simulink model "F2sidecarv4"  (R2018b)
settings: Solver=ode45  StartTime=0.0  StopTime=20  MaxStep=1e-3  RelTol=1e-5
values from neighbouring files (symbols this model uses):
  g = 9.8    [GG.m]    (also in main.m)
  HGC = 0.165    [main.m]
  Iz = 80    [main.m]
  lf = 0.7    [main.m]
  lr = WB-lf    (= 0.6)    [main.m]
  ls = lr-lshift    (= 0.6)    [main.m]
  lshift = 0.2    [main.m]
  m = 180    [main.m]
  TrackL = 0.7*Track    (= 0.7735)    [main.m]
  TrackRf = TrackRr-frontwheel_shift    (= 0.3315)    [main.m]
  TrackRr = Track-TrackL    (= 0.3315)    [main.m]
  v0 = 20    [main.m]
  WB = 1.2    [main.m]
libraries: simulink x5
settings Model: Creator=PHADM  LastModifiedBy=PHADM
settings SolverCC: AlgebraicLoopSolver=LineSearch

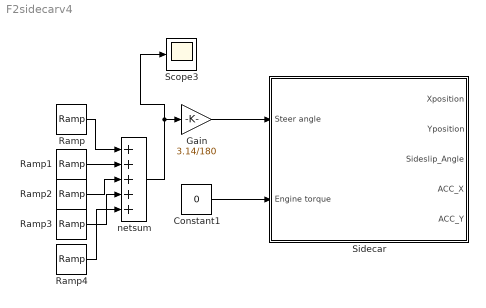
== system F2sidecarv4 ==
  Constant1 : Constant  Value=0
  Gain : Gain  Gain=3.14/180
  Ramp : simulink/Sources/Ramp  slope=-10  start=0  InitialOutput=0
  Ramp1 : simulink/Sources/Ramp  slope=10  start=2  InitialOutput=0
  Ramp2 : simulink/Sources/Ramp  slope=0  start=3  InitialOutput=0
  Ramp3 : simulink/Sources/Ramp  slope=0  start=8  InitialOutput=0
  Ramp4 : simulink/Sources/Ramp  slope=0  start=10  InitialOutput=0
  Scope3 : Scope
  "Sidecar " : Subsystem
  netsum : Sum  Inputs=5  SaturateOnIntegerOverflow=on  InputSameDT=on  OutDataTypeStr=Inherit: Same as first input
  wires:
  Constant1/1 -> "Sidecar "/2(Engine torque)
  Gain/1 -> "Sidecar "/1("Steer angle ")
  Ramp/1 -> netsum/1
  netsum/1 -> Scope3/1, Gain/1
  Ramp1/1 -> netsum/2
  Ramp2/1 -> netsum/3
  Ramp3/1 -> netsum/4
  Ramp4/1 -> netsum/5

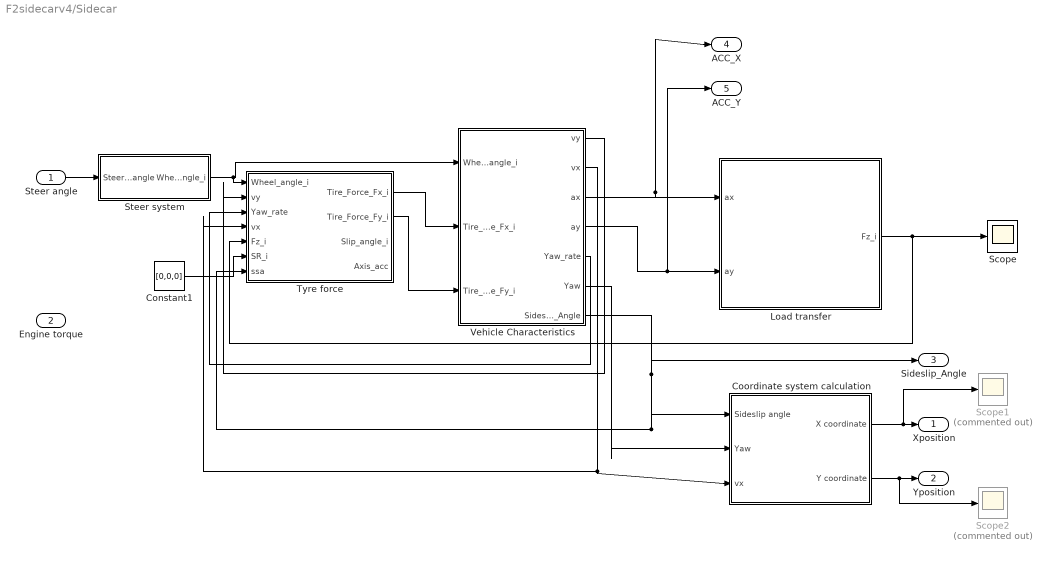
== system F2sidecarv4/Sidecar  ==
  "Steer angle " : Inport
  Engine torque : Inport  Port=2
  Constant1 : Constant  Value=[0,0,0]
  Coordinate system calculation : Subsystem
  Load transfer : Subsystem
  Scope : Scope
  Scope1 : Scope  Commented=on
  Scope2 : Scope  Commented=on
  Steer system : Subsystem
  Tyre force : Subsystem
  Vehicle Characteristics : Subsystem
  Xposition : Outport
  Yposition : Outport  Port=2
  Sideslip_Angle : Outport  Port=3
  ACC_X : Outport  Port=4
  ACC_Y : Outport  Port=5
  wires:
  Steer system/1(Wheel_angle_i) -> Vehicle Characteristics/1(Wheel_angle_i), Tyre force/1(Wheel_angle_i)
  Vehicle Characteristics/3(ax) -> ACC_X/1, Load transfer/1(ax)
  Vehicle Characteristics/4(ay) -> ACC_Y/1, Load transfer/2(ay)
  Vehicle Characteristics/6(Yaw) -> Coordinate system calculation/2(Yaw)
  Vehicle Characteristics/2(vx) -> Tyre force/4(vx), Coordinate system calculation/3(vx)
  Coordinate system calculation/1(X coordinate) -> Scope1/1, Xposition/1
  Coordinate system calculation/2(Y coordinate) -> Scope2/1, Yposition/1
  Tyre force/1(Tire_Force_Fx_i) -> Vehicle Characteristics/2("Tire_Force_Fx_i ")
  Tyre force/2(Tire_Force_Fy_i) -> Vehicle Characteristics/3(Tire_Force_Fy_i)
  Constant1/1 -> Tyre force/6(SR_i)
  Vehicle Characteristics/5(Yaw_rate) -> Tyre force/3(Yaw_rate)
  Vehicle Characteristics/7(Sideslip_Angle) -> Coordinate system calculation/1(Sideslip angle), Tyre force/7(ssa), Sideslip_Angle/1
  Load transfer/1(Fz_i) -> Tyre force/5(Fz_i), Scope/1
  Vehicle Characteristics/1(vy) -> Tyre force/2(vy)
  "Steer angle "/1 -> Steer system/1(Steer_angle)

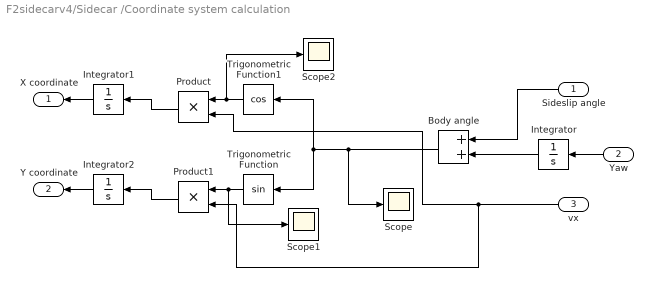
== system F2sidecarv4/Sidecar /Coordinate system calculation ==
  Sideslip angle : Inport
  Yaw : Inport  Port=2
  vx : Inport  Port=3
  Body angle : Sum
  Integrator : Integrator
  Integrator1 : Integrator
  Integrator2 : Integrator
  Product : Product
  Product1 : Product
  Scope : Scope
  Scope1 : Scope
  Scope2 : Scope
  Trigonometric Function : Trigonometry
  Trigonometric Function1 : Trigonometry  Operator=cos
  X coordinate : Outport
  Y coordinate : Outport  Port=2
  wires:
  vx/1 -> Product/2, Product1/2
  Yaw/1 -> Integrator/1
  Sideslip angle/1 -> Body angle/1
  Integrator2/1 -> Y coordinate/1
  Integrator1/1 -> X coordinate/1
  Product1/1 -> Integrator2/1
  Product/1 -> Integrator1/1
  Trigonometric Function/1 -> Scope1/1, Product1/1
  Trigonometric Function1/1 -> Product/1, Scope2/1
  Body angle/1 -> Scope/1, Trigonometric Function1/1, Trigonometric Function/1
  Integrator/1 -> Body angle/2

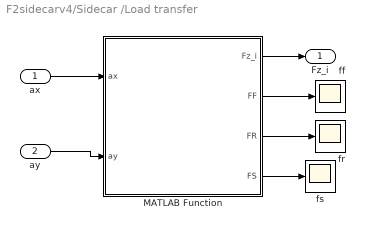
== system F2sidecarv4/Sidecar /Load transfer ==
  ax : Inport
  ay : Inport  Port=2
  MATLAB Function : MATLAB Function  TreatAsAtomicUnit=on
  ff : Scope
  fr : Scope
  fs : Scope
  Fz_i : Outport
  wires:
  MATLAB Function/1(Fz_i) -> Fz_i/1
  ax/1 -> MATLAB Function/1(ax)
  ay/1 -> MATLAB Function/2(ay)
  MATLAB Function/4(FS) -> fs/1
  MATLAB Function/3(FR) -> fr/1
  MATLAB Function/2(FF) -> ff/1

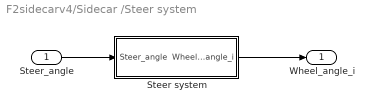
== system F2sidecarv4/Sidecar /Steer system ==
  Steer_angle : Inport
  Steer system : MATLAB Function  TreatAsAtomicUnit=on
  Wheel_angle_i : Outport
  wires:
  Steer_angle/1 -> Steer system/1(Steer_angle)
  Steer system/1(Wheel_angle_i) -> Wheel_angle_i/1

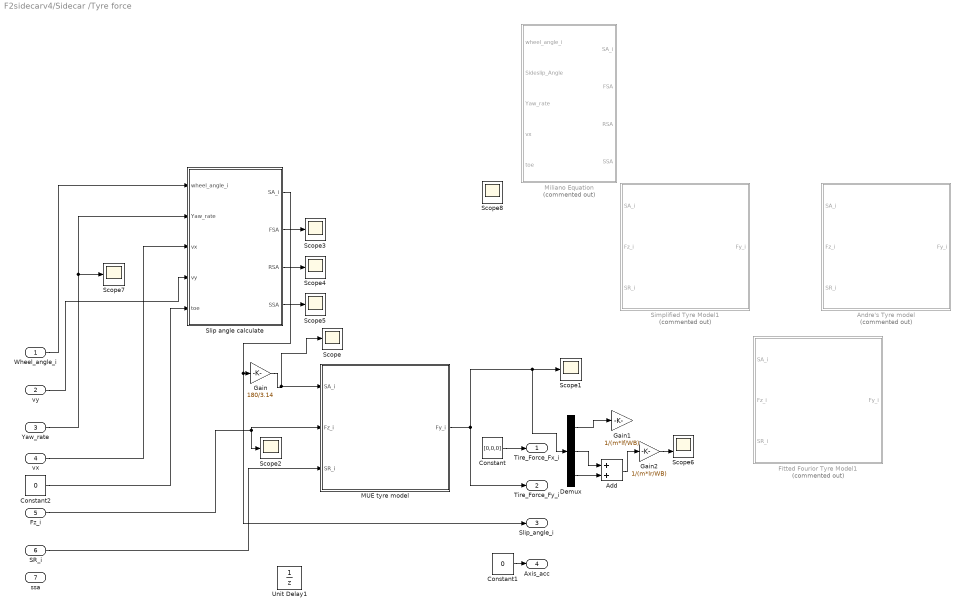
== system F2sidecarv4/Sidecar /Tyre force ==
  Wheel_angle_i : Inport
  vy : Inport  Port=2
  Yaw_rate : Inport  Port=3
  vx : Inport  Port=4
  Fz_i : Inport  Port=5
  SR_i : Inport  Port=6
  ssa : Inport  Port=7
  Add : Sum
  Andre's Tyre model : MATLAB Function  Commented=on  TreatAsAtomicUnit=on
  Constant : Constant  Value=[0,0,0]
  Constant1 : Constant  Value=0
  Constant2 : Constant  Value=0
  Demux : Demux  Outputs=3
  Fitted Fourior Tyre Model1 : MATLAB Function  Commented=on  TreatAsAtomicUnit=on
  Gain : Gain  Gain=180/3.14
  Gain1 : Gain  Gain=1/(m*lf/WB)
  Gain2 : Gain  Gain=1/(m*lr/WB)
  MUE tyre model : MATLAB Function  TreatAsAtomicUnit=on
  Miliano Equation : MATLAB Function  Commented=on  TreatAsAtomicUnit=on
  Scope{,1..5,7..8} (8 alike) : Scope
  Scope6 : Scope  NumInputPorts=2
  Simplified Tyre Model1 : MATLAB Function  Commented=on  TreatAsAtomicUnit=on
  Slip angle calculate : MATLAB Function  TreatAsAtomicUnit=on
  Unit Delay1 : UnitDelay  SampleTime=-1
  Tire_Force_Fx_i : Outport
  Tire_Force_Fy_i : Outport  Port=2
  Slip_angle_i : Outport  Port=3
  Axis_acc : Outport  Port=4
  wires:
  Wheel_angle_i/1 -> Slip angle calculate/1(wheel_angle_i)
  vy/1 -> Slip angle calculate/4(vy)
  Yaw_rate/1 -> Slip angle calculate/2(Yaw_rate), Scope7/1
  vx/1 -> Slip angle calculate/3(vx)
  Constant/1 -> Tire_Force_Fx_i/1
  Constant1/1 -> Axis_acc/1
  SR_i/1 -> MUE tyre model/3(SR_i)
  MUE tyre model/1(Fy_i) -> Demux/1, Scope1/1, Tire_Force_Fy_i/1
  Constant2/1 -> Slip angle calculate/5(toe)
  Slip angle calculate/2(FSA) -> Scope3/1
  Slip angle calculate/3(RSA) -> Scope4/1
  Slip angle calculate/4(SSA) -> Scope5/1
  Fz_i/1 -> MUE tyre model/2(Fz_i), Scope2/1
  Gain/1 -> MUE tyre model/1(SA_i), Scope/1
  Demux/1 -> Gain1/1
  Demux/2 -> Add/1
  Gain2/1 -> Scope6/2
  Demux/3 -> Add/2
  Add/1 -> Gain2/1
  Slip angle calculate/1(SA_i) -> Slip_angle_i/1, Gain/1

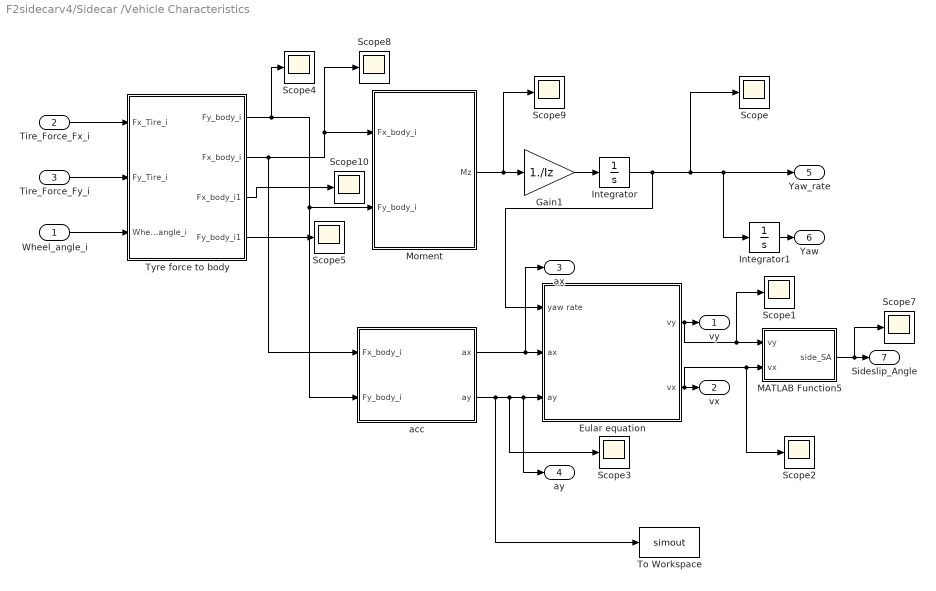
== system F2sidecarv4/Sidecar /Vehicle Characteristics ==
  Wheel_angle_i : Inport
  "Tire_Force_Fx_i " : Inport  Port=2
  Tire_Force_Fy_i : Inport  Port=3
  Eular equation : Subsystem
  Gain1 : Gain  Gain=1./Iz
  Integrator : Integrator
  Integrator1 : Integrator
  MATLAB Function5 : MATLAB Function  TreatAsAtomicUnit=on
  Moment : MATLAB Function  TreatAsAtomicUnit=on
  Scope{,1..5,7..10} (10 alike) : Scope
  To Workspace : ToWorkspace  VariableName=simout  SaveFormat=Timeseries  SampleTime=-1
  Tyre force to body : Subsystem
  acc : MATLAB Function  TreatAsAtomicUnit=on
  vy : Outport
  vx : Outport  Port=2
  ax : Outport  Port=3
  ay : Outport  Port=4
  Yaw_rate : Outport  Port=5
  Yaw : Outport  Port=6
  Sideslip_Angle : Outport  Port=7
  wires:
  Wheel_angle_i/1 -> Tyre force to body/3(Wheel_angle_i)
  Tire_Force_Fy_i/1 -> Tyre force to body/2(Fy_Tire_i)
  "Tire_Force_Fx_i "/1 -> Tyre force to body/1(Fx_Tire_i)
  Moment/1(Mz) -> Scope9/1, Gain1/1
  Gain1/1 -> Integrator/1
  Integrator/1 -> Eular equation/1(yaw rate), Integrator1/1, Yaw_rate/1, Scope/1
  Integrator1/1 -> Yaw/1
  acc/1(ax) -> ax/1, Eular equation/2(ax)
  acc/2(ay) -> To Workspace/1, Scope3/1, ay/1, Eular equation/3(ay)
  Eular equation/1(vy) -> Scope1/1, MATLAB Function5/1(vy), vy/1
  Eular equation/2(vx) -> Scope2/1, MATLAB Function5/2(vx), vx/1
  MATLAB Function5/1(side_SA) -> Scope7/1, Sideslip_Angle/1
  Tyre force to body/1(Fy_body_i) -> Scope4/1, acc/2(Fy_body_i), Moment/2(Fy_body_i)
  Tyre force to body/4(Fy_body_i1) -> Scope5/1
  Tyre force to body/2(Fx_body_i) -> acc/1(Fx_body_i), Moment/1(Fx_body_i), Scope8/1
  Tyre force to body/3(Fx_body_i1) -> Scope10/1

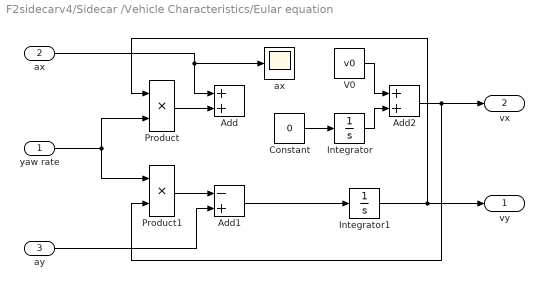
== system F2sidecarv4/Sidecar /Vehicle Characteristics/Eular equation ==
  yaw rate : Inport
  ax : Inport  Port=2
  ay : Inport  Port=3
  Add : Sum
  Add1 : Sum  Inputs=-+
  Add2 : Sum
  Constant : Constant  Value=0
  Integrator : Integrator  LimitOutput=on  LowerSaturationLimit=0  IgnoreLimit=on
  Integrator1 : Integrator  LowerSaturationLimit=0  IgnoreLimit=on
  Product : Product
  Product1 : Product
  V0 : Constant  Value=v0
  "ax " : Scope
  vy : Outport
  vx : Outport  Port=2
  wires:
  yaw rate/1 -> Product/2, Product1/1
  ax/1 -> "ax "/1, Add/1
  Add1/1 -> Integrator1/1
  Integrator/1 -> Add2/2
  Product1/1 -> Add1/1
  ay/1 -> Add1/2
  Constant/1 -> Integrator/1
  V0/1 -> Add2/1
  Integrator1/1 -> vy/1, Product/1
  Product/1 -> Add/2
  Add2/1 -> Product1/2, vx/1

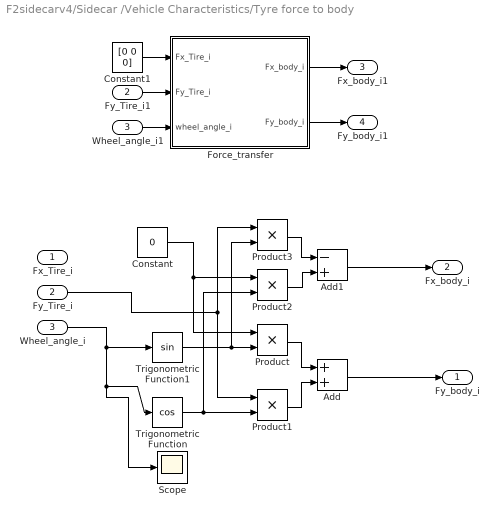
== system F2sidecarv4/Sidecar /Vehicle Characteristics/Tyre force to body ==
  Fx_Tire_i : Inport
  Fy_Tire_i : Inport  Port=2
  Wheel_angle_i : Inport  Port=3
  Add : Sum
  Add1 : Sum  Inputs=-+
  Constant : Constant  Value=0
  Constant1 : Constant  Value=[0 0 0]
  Force_transfer : MATLAB Function  TreatAsAtomicUnit=on
  Fy_Tire_i1 : InportShadow  Port=2
  Product{,1..3} (4 alike) : Product
  Scope : Scope
  Trigonometric Function : Trigonometry  Operator=cos  ApproximationMethod=CORDIC
  Trigonometric Function1 : Trigonometry  ApproximationMethod=CORDIC
  Wheel_angle_i1 : InportShadow  Port=3
  Fy_body_i : Outport
  Fx_body_i : Outport  Port=2
  Fx_body_i1 : Outport  Port=3
  Fy_body_i1 : Outport  Port=4
  wires:
  Constant/1 -> Product/1, Product2/1
  Product2/1 -> Add1/2
  Product3/1 -> Add1/1
  Product1/1 -> Add/2
  Product/1 -> Add/1
  Fy_Tire_i/1 -> Product1/1, Product3/1
  Trigonometric Function/1 -> Product1/2, Product2/2
  Trigonometric Function1/1 -> Product/2, Product3/2
  Wheel_angle_i/1 -> Scope/1, Trigonometric Function/1, Trigonometric Function1/1
  Add1/1 -> Fx_body_i/1
  Add/1 -> Fy_body_i/1
  Force_transfer/2(Fy_body_i) -> Fy_body_i1/1
  Force_transfer/1(Fx_body_i) -> Fx_body_i1/1
  Fy_Tire_i1/1 -> Force_transfer/2(Fy_Tire_i)
  Constant1/1 -> Force_transfer/1(Fx_Tire_i)
  Wheel_angle_i1/1 -> Force_transfer/3(wheel_angle_i)

== matlab function F2sidecarv4/Sidecar /Tyre force/Fitted Fourior Tyre Model1 ==
  data: SA_i input size=3; Fy_i output size=3; Fz_i input size=3; SR_i input size=3
function Fy_i = fcn(SA_i,Fz_i,SR_i)
SR_i=[0,0,0];
Fy_i=zeros(3,1);
Fy_i0=zeros(3,1);


i=1;
while i<4
    if SA_i(i)>10
    SA_i(i)=10;
else if SA_i(i)<-10
        SA_i(i)=-10;
    end
end
Fy_i0(i)=  -85.64 + 115*cos(SA_i(i)*0.3621) + 1640*sin(SA_i(i)*0.3621) + (-117.5)*cos(2*SA_i(i)*0.3621) + (-158.2)*sin(2*SA_i(i)*0.3621) + 70.39*cos(3*SA_i(i)*0.3621) + 221.5*sin(3*SA_i(i)*0.3621) +(-50.6)*cos(4*SA_i(i)*0.3621) + (-14.42)*sin(4*SA_i(i)*0.3621) + 19.82*cos(5*SA_i(i)*0.3621) + 20.98*sin(5*SA_i(i)*0.3621) + (-8.731)*cos(6*SA_i(i)*0.3621) + 9.067*sin(6*SA_i(i)*0.3621);
Fy_i(i)=0.65*Fy_i0(i);
i=i+1;
end
end

== matlab function F2sidecarv4/Sidecar /Tyre force/Miliano Equation ==
  data: wheel_angle_i input; SA_i output; Sideslip_Angle input; Yaw_rate input; vx input; FSA output; RSA output; SSA output; lf parameter; lr parameter; lshift parameter; TrackL parameter; TrackRf parameter; toe input; TrackRr parameter
%%TrackL+TrackR=Track
%%lr+lf=Wheel base
%%ls-distance gravity centre to sidewheel
function [SA_i,FSA,RSA,SSA] = fcn(wheel_angle_i,Sideslip_Angle,Yaw_rate,vx,lf, lr, lshift, TrackL, TrackRf,toe, TrackRr)
SA_i=zeros(3,1);

SA_i(1)=atan(((vx*tan(Sideslip_Angle)+Yaw_rate*lf)*cos(wheel_angle_i(1))-((vx-Yaw_rate*TrackRf)*cos(wheel_angle_i(1))))/((vx-Yaw_rate*TrackRf)*cos(wheel_angle_i(1))+(vx*tan(Sideslip_Angle)+Yaw_rate*lf)*sin(wheel_angle_i(1)))); %%front wheel(right)
SA_i(2)=atan((vx*tan(Sideslip_Angle)-Yaw_rate*lr)/(vx+Yaw_rate*TrackRr));%%rear wheel(right)
SA_i(3)=atan(((vx*tan(Sideslip_Angle)-Yaw_rate*(lshift))*cos(toe)-(vx-Yaw_rate*(TrackL))*sin(toe))/(vx-Yaw_rate*(TrackL)*cos(toe)+(vx*tan(Sideslip_Angle)+Yaw_rate*(lshift)))); %%side wheel(left)

FSA=SA_i(1);
RSA=SA_i(2);
SSA=SA_i(3);
end

== matlab function F2sidecarv4/Sidecar /Steer system/Steer system ==
  data: Steer_angle input; Wheel_angle_i output
function Wheel_angle_i  = fcn(Steer_angle)
Wheel_angle_i=zeros(3,1);
Wheel_angle_i(1) = Steer_angle;
Wheel_angle_i(2)=0;
Wheel_angle_i(3)=0;
end

== matlab function F2sidecarv4/Sidecar /Vehicle Characteristics/Moment ==
  data: Fx_body_i input size=3; Mz output; Fy_body_i input size=3; lf parameter; lr parameter; ls parameter; TrackL parameter; TrackRf parameter; TrackRr parameter
function Mz = fcn(Fx_body_i,Fy_body_i,lf, lr, ls, TrackL, TrackRf,TrackRr)
Mz=zeros(1,1);
Mz=Fy_body_i(1).*lf-Fy_body_i(2).*lr-Fy_body_i(3).*ls+TrackRf*(-(Fx_body_i(1)))+TrackRr*(-(Fx_body_i(2))+TrackL*(Fx_body_i(3)));
end

== matlab function F2sidecarv4/Sidecar /Vehicle Characteristics/acc ==
  data: Fx_body_i input size=3; ax output; Fy_body_i input size=3; ay output; m parameter
function [ax,ay] = fcn(Fx_body_i,Fy_body_i,m)

ax=(Fx_body_i(1)+Fx_body_i(2)+Fx_body_i(3))/m;
ay=(Fy_body_i(1)+Fy_body_i(2)+Fy_body_i(3))/m;
end

== matlab function F2sidecarv4/Sidecar /Vehicle Characteristics/Tyre force to body/Force_transfer ==
  data: Fx_Tire_i input size=3; Fx_body_i output size=3; Fy_Tire_i input size=3; wheel_angle_i input size=3; Fy_body_i output size=3
function [Fx_body_i,Fy_body_i] = fcn(Fx_Tire_i,Fy_Tire_i,wheel_angle_i)
Fy_body_i=ones(3,1);
Fx_body_i=ones(3,1);
    Fy_body_i(1)=sin(wheel_angle_i(1)).*Fx_Tire_i(1)+cos(wheel_angle_i(1)).*Fy_Tire_i(1);
    Fy_body_i(2)=sin(wheel_angle_i(2)).*Fx_Tire_i(2)+cos(wheel_angle_i(2)).*Fy_Tire_i(2);
    Fy_body_i(3)=sin(wheel_angle_i(3)).*Fx_Tire_i(3)+cos(wheel_angle_i(3)).*Fy_Tire_i(3); 
    Fx_body_i(1)=cos(wheel_angle_i(1)).*Fx_Tire_i(1)-sin(wheel_angle_i(1)).*Fy_Tire_i(1);
    Fx_body_i(2)=cos(wheel_angle_i(2)).*Fx_Tire_i(2)-sin(wheel_angle_i(2)).*Fy_Tire_i(2);
    Fx_body_i(3)=cos(wheel_angle_i(3)).*Fx_Tire_i(3)-sin(wheel_angle_i(3)).*Fy_Tire_i(3);
end

== matlab function F2sidecarv4/Sidecar /Load transfer/MATLAB Function ==
  data: ax input; Fz_i output; ay input; TrackL parameter; TrackRf parameter; TrackRr parameter; lf parameter; lr parameter; m parameter; HGC parameter; lshift parameter; g parameter; ls parameter; FF output; FR output; FS output
function [Fz_i,FF,FR,FS]  = fcn(ax,ay,TrackL,TrackRf,TrackRr, lf, lr, m,HGC, lshift, g, ls)
Fz_i=zeros(3,1);
%%%Calculate equation
%Fz_i(1)+Fz_i(2)+Fz_i(3)=m*g
%Fz_i(1)*WB+Fz_i(3)*(lr-lshift)=m*g*WB+m*ax*HGC
%Fz_i(3)*Track=m*g*TrackR+m*ay*HGC

%%%Matrix
left=[1 1 1
      -lf lr ls
      -TrackRf -TrackRr TrackL
      ];
right=[m*g
     m*ax*HGC
     m*ay*HGC
     ];
 
Fz_i=inv(left)*right;
for i=1:3
if Fz_i(i)<0
    Fz_i(i)=0;
end

end
FF=Fz_i(1);
FR=Fz_i(2);
FS=Fz_i(3);
end

== matlab function F2sidecarv4/Sidecar /Tyre force/Slip angle calculate ==
  data: wheel_angle_i input; Yaw_rate input; vx input; SA_i output; vy input; FSA output; RSA output; SSA output; lf parameter; lr parameter; ls parameter; TrackL parameter; TrackRf parameter; TrackRr parameter; toe input
%%TrackL+TrackR=Track
%%lr+lf=Wheel base
%%ls-distance gravity centre to sidewheel
%1-front wheel
%2-rear wheel
%3-side wheel
function [SA_i,FSA,RSA,SSA] = slipangle(wheel_angle_i,Yaw_rate,vx,vy,lf, lr, ls, TrackL, TrackRf,TrackRr,toe)
SA_i=zeros(3,1);

% SA_i(1)=wheel_angle_i(1)-(Sideslip_Angle+atan(lf*Yaw_rate/(vx)));%%front wheel(right)
% SA_i(2)=-(Yaw_rate*lr/(vx)+Sideslip_Angle);%%rear wheel(right)
% SA_i(3)=-(Yaw_rate*ls/(vx)+Sideslip_Angle);%%side wheel(left)
% SA_i(1)=wheel_angle_i(1)-atan((lf*Yaw_rate+vy)/(vx-TrackRf*Yaw_rate));
SA_i(1)=((vy+Yaw_rate*lf)*cos(wheel_angle_i(1))-(vx-Yaw_rate*TrackRf)*sin(wheel_angle_i(1)))/((vx-Yaw_rate*TrackRf)*cos(wheel_angle_i(1))+(vy+Yaw_rate*lf)*sin(wheel_angle_i(1)));
SA_i(2)=(Yaw_rate*lr-vy)/(vx-TrackRr*Yaw_rate);
SA_i(3)=(Yaw_rate*ls-vy)/(vx+TrackL*Yaw_rate);

FSA=SA_i(1);
RSA=SA_i(2);
SSA=SA_i(3);
end

== matlab function F2sidecarv4/Sidecar /Tyre force/Andre's Tyre model ==
  data: SA_i input size=3; Fy_i output size=3; Fz_i input size=3; SR_i input size=3
function Fy_i = fcn(SA_i,Fz_i,SR_i)
SR_i=[0,0,0];
Fy_i=zeros(3,1);

p1=zeros(3,1);
p2=zeros(3,1);
p3=zeros(3,1);
p4=zeros(3,1);
i=1;
while i<4
if Fz_i(i)>840 && Fz_i(i)<=1050
       p1(i) =        11.4;
       p2(i) =      -109.3;  
       p3(i) =       207.7;  
       p4(i) =         601;
else if Fz_i(i)>1050 && Fz_i(i)<=1260
       p1(i)=       13.86;
       p2(i) =      -134.5;
       p3(i)=       270.5;
       p4(i)=       657.7;
    else if Fz_i(i)>1260 && Fz_i(i)<=1470
       p1(i) =       15.03;
       p2(i) =      -146.3;
       p3(i) =       295.2;
       p4(i) =       730.1;
        else if Fz_i(i)>1470
       p1(i) =       9.707;
       p2(i) =      -89.29;
       p3(i) =       103.7;
       p4(i) =       979.1;
            else if Fz_i(i)<840 && Fz_i(i)>00
       p1(i) =       9.071;
       p2(i) =      -86.06;
       p3(i) =       154.7;
       p4(i) =       517.4;
                else if Fz_i(i)<=0
       p1(i) =       0;
       p2(i) =       0;
       p3(i) =       0;
       p4(i) =       0;
                    end
                end
            end
        end
    end
end
Cs= p1(i).*SA_i(i)^3 + p2(i).*SA_i(i)^2 + p3(i).*SA_i(i) + p4(i);
Fy_i(i)=Cs.*SA_i(i)*0.65;
i=i+1;
end
          
end

== matlab function F2sidecarv4/Sidecar /Tyre force/Simplified Tyre Model1 ==
  data: SA_i input size=3; Fy_i output size=3; Fz_i input size=3; SR_i input size=3
function Fy_i = fcn(SA_i,Fz_i,SR_i)
SR_i=[0,0,0];
Fy_i=zeros(3,1);

p1=zeros(3,1);
p2=zeros(3,1);
p3=zeros(3,1);
p4=zeros(3,1);
i=1;
while i<4
if SA_i(i)>=0
if Fz_i(i)>0
       p1(i) =       9.071;
       p2(i) =      -86.06;
       p3(i) =       154.7;
       p4(i) =       517.4;
    else if Fz_i(i)<=0
       p1(i) =       0;
       p2(i) =       0;
       p3(i) =       0;
       p4(i) =       0;

    end
end
Cs= p1(i).*SA_i(i)^3 + p2(i).*SA_i(i)^2 + p3(i).*SA_i(i) + p4(i);
Fy_i(i)=Cs.*SA_i(i)*0.65;
    else 
        SA_i(i)=abs(SA_i(i));
if  Fz_i(i)>0
       p1(i) =       9.071;
       p2(i) =      -86.06;
       p3(i) =       154.7;
       p4(i) =       517.4;
    else if Fz_i(i)<=0
       p1(i) =       0;
       p2(i) =       0;
       p3(i) =       0;
       p4(i) =       0;
 
         end
end
Cs= p1(i).*SA_i(i)^3 + p2(i).*SA_i(i)^2 + p3(i).*SA_i(i) + p4(i);
Fy_i(i)=-Cs.*SA_i(i)*0.65;
    end
i=i+1;
end
          
end

== matlab function F2sidecarv4/Sidecar /Tyre force/MUE tyre model ==
  data: SA_i input size=3; Fy_i output size=3; Fz_i input size=3; SR_i input size=3
function Fy_i = fcn(SA_i,Fz_i,SR_i)
SR_i=[0,0,0];
Fy_i=zeros(3,1);
Fy_i0=zeros(3,1);


i=1;
while i<4
%     if Fz_i(i)<=840.9
%     mumaxy=(Fz_i(i)-0)*(1.806934-0)/(840.9-0)+1.806934;
%     muy=mumaxy*sin(1.3*atan(3.1415926/2/atan(1.3)*SA_i(i)/5.74));
%     Fy_i(i)=Fz_i(i)*muy;
%     else if Fz_i(i)>840.9 && Fz_i(i)<=1051
    mumaxy=(Fz_i(i)-840.9)*(1.754256934-1.806934)/(1051-840.9)+1.806934;
    muy=mumaxy*sin(1.3*atan(3.1415926/2/atan(1.3)*SA_i(i)/5.74));
    Fy_i(i)=Fz_i(i)*muy;
            if Fz_i(i)>1051 && Fz_i(i)<=1261
            mumaxy=(Fz_i(i)-1051)*(1.684838-1.754257)/(1261-1051)+1.754257;
            muy=mumaxy*sin(1.3*atan(3.1415926/2/atan(1.3)*SA_i(i)/5.74));
            Fy_i(i)=Fz_i(i)*muy;
                    else if Fz_i(i)>1261 && Fz_i(i)<=1471
                    mumaxy=(Fz_i(i)-1261)*(1.607952-1.684838)/(1471-1261)+1.684838;
                    muy=mumaxy*sin(1.3*atan(3.1415926/2/atan(1.3)*SA_i(i)/5.74));
                    Fy_i(i)=Fz_i(i)*muy;
                            else if Fz_i(i)>1471
                            mumaxy=(Fz_i(i)-1471)*(1.5624-1.607952)/(1681-1471)+1.607952;
                            muy=mumaxy*sin(1.3*atan(3.1415926/2/atan(1.3)*SA_i(i)/5.74));
                            Fy_i(i)=Fz_i(i)*muy;

%                                 end
                        end
                end
            end
            i=i+1;
    end
       
end

== matlab function F2sidecarv4/Sidecar /Vehicle Characteristics/MATLAB Function5 ==
  data: vy input; vx input; side_SA output
function side_SA  = fcn(vy,vx)
%#codegen

side_SA=atan(vy./vx);
end
